simulink library "taXlibrary"  (Simulink 8.6)
settings: Solver=ode45  StartTime=0.0  StopTime=10.0  RelTol=1e-3
undefined symbols (not defined in the file): data, model, observer, scatteringDummy, sys, triJunction_12
settings Model: Creator=mur  LastModifiedBy=jaensch

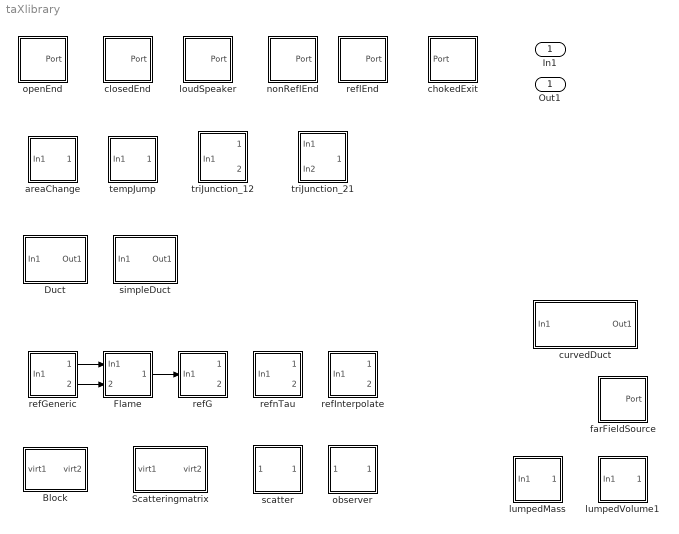
== system taXlibrary ==
  In1 : Inport
  Block : Subsystem  mask{element=Element, nIn=1, nOut=1, filename=/home/thomas/tools/taX/Projects/Orifice_Carlo/L0D_Element.mat, modelname=sys}
      mask prompts: nIn "Number of input ports"; nOut "Number of output ports"
      mask init:
      | % Set identifier
      | set_param(gcb,'element',char('Element'));
      | 
      | adaptIO(gcb);
      mask Display:
      | text(.3, .3, 'S21', 'HorizontalAlignment', 'center')
      | text(.3, .7, 'S11', 'HorizontalAlignment', 'center')
      | text(.7, .3, 'S22', 'HorizontalAlignment', 'center')
      | text(.7, .7, 'S12', 'HorizontalAlignment', 'center')
      | plot([.2 .1 .1 .2], [.9 .9 .1 .1])
      | plot([.8 .9 .9 .8], [.9 .9 .1 .1])
      | %plot([1 1 0 0 1],[1 0 0 1 1])
  Duct : Subsystem  mask{element=Duct, order=3, minres=40, l=0.5, sensorPositions=[]}
      mask prompts: order "Order of upwind scheme"; minres "Resolution of shortest wave"; l "Length [m]"; sensorPositions "Sensor Positions [m]"
      mask init:
      | % Set identifier
      | set_param(gcb,'element',char('Duct'));
      settings: AttributesFormatString=%<l> m
      mask TypeOptions order: 1 | 2 | 3 | inf
      mask Display:
      | patch([0 1 1 0],[.2 .2 .8 .8],[.7 1 1])
      | plot([0 1],[.2 .2])
      | plot([0 1],[.8 .8])
      | 
      | plot([1 1 0 0 1],[1 0 0 1 1])
  Flame : Subsystem  mask{element=rankineHugoniot, nRef=1, Mach=0.001056*101325/(287.04*293)*11.3/(101325/(287.04*1930)*0.0081*sqrt(1.4*287.04*1930)), rho=101325/(287.04*1930), c=sqrt(1.4*287.04*1930)}
      mask prompts: nRef "Number of heat release fluctuation references"; Mach "Mach number [-]"; rho "Density [Kg/m³]"; c "Speed of sound [m/s]"
      mask init:
      | set_param(gcb,'element',char('rankineHugoniot'));
      | 
      | switchNRef(gcb,nRef);
      mask Display:
      | plot([-.1 1.1], [.5 .5])
      | %patch([-.1 1.1 1.1 -.1],[-.1 -.1 1.1 1.1],[.7 1 1])
      | patch([.3 .4 .3 .4 .3 .4 .3 .4 .3 .4 .3 ...
      |        .5 .8 .5 .8 .5 .8 .5 .8 .5 .8 .5],...
      |       [ 1 .9 .8 .7 .6 .5 .4 .3 .2 .1 0 ...
      |         0 .1 .2 .3 .4 .5 .6 .7 .8 .9 1 ],[1 .75 0])
      | 
      | color('red')
      | plot([.3 .4 .3 .4 .3 .4 .3 .4 .3 .4 .3],...
      |      [ 0 .1 .2 .3 .4 .5 .6 .7 .8 .9  1])
      | plot([.4 .6 .4 .6 .4 .6 .4 .6 .4 .6 .4],...
      |      [ 0 .1 .2 .3 .4 .5 .6 .7 .8 .9  1])
      | plot([.3 .5 .8 .5 .8 .5 .8 .5 .8 .5 .8 .5 .3],...
      |      [ 0  0 .1 .2 .3 .4 .5 .6 .7 .8 .9  1  1])
  Scatteringmatrix : Subsystem  mask{element=ScatteringMatrix, filename=/home/thomas/Data/MeindlComsol/Duct/ducttest.mat, modelname=sys, l=1, A=[1], Mach=[2.2204e-18], rho=[1.3], c=[100]}
      mask prompts: l "Length [m]"; A "Area [m²]"; Mach "Mach number [-]"; rho "Density [Kg/m³]"; c "Speed of sound [m/s]"
      mask init:
      | % Set identifier
      | set_param(gcb,'element',char('ScatteringMatrix'));
      | 
      | adaptScatterIO(gcb);
      settings: AttributesFormatString=%<modelname>
      mask Display:
      | text(.3, .3, 'S21', 'HorizontalAlignment', 'center')
      | text(.3, .7, 'S11', 'HorizontalAlignment', 'center')
      | text(.7, .3, 'S22', 'HorizontalAlignment', 'center')
      | text(.7, .7, 'S12', 'HorizontalAlignment', 'center')
      | plot([.2 .1 .1 .2], [.9 .9 .1 .1])
      | plot([.8 .9 .9 .8], [.9 .9 .1 .1])
      | %plot([1 1 0 0 1],[1 0 0 1 1])
  areaChange : Subsystem  mask{element=lZeta, zeta=0, lred=0, leff=0, l=1, A=4}
      mask prompts: zeta "Pressure loss Coefficient zeta"; lred "Reduced Length l_red"; leff "Effective Length l_eff"; l "Length [m]"; A "Area [m²]"
      mask init:
      | % Set identifier
      | set_param(gcb,'element',char('lZeta'));
      settings: AttributesFormatString=%<A> m²
      mask Display:
      | patch([0 0 .6 .6  1  1 .6 .6 0], ...
      |       [.1 .9  .9 .7 .7 .3 .3  0.1 0.1], ...
      |       [.7 1 1])
      | 
      | % plot([0   0    .1 .2  .3 .4  .5 .6 .6 1   1   .6 .6  .5 .4 .3 .2  .1 0  ], ...
      | %      [ .1  .9 1   .9 1   .9 1   .9 .7  .7  .3 .3 .1 0   .1 0 .1 0    .1])
      | 
      | plot([0 .6 .6 1 1 .6 .6 0], ...
      |      [.9 .9 .7 .7 .3 .3 .1 .1])
      | 
      | plot([0 1 1 0 0], ...
      |      [1 1 0 0 1])
      | 
      | text(.3,.5,'L','HorizontalAlignment','center')
      | text(.6,.5,'zt','HorizontalAlignment','center')
  chokedExit : Subsystem  mask{element=chokedExit, loc=Downstream, Gamma=1.4, A=1, Mach=0.1, rho=1, c=100}
      mask prompts: loc "Location"; Gamma "Gamma [-]"; A "Area [m²]"; Mach "Mach number"; rho "Density [kg/m³]"; c "Speed of sound [m/s]"
      mask init:
      | % Set identifier
      | set_param(gcb,'element',char('chokedExit'));
      | 
      | switchBCUpDownStream(gcb,loc);
      mask TypeOptions loc: Downstream | Upstream
      mask Display:
      | patch([0 .5 .5 0],[.2 .2 .8 .8],[.7 1 1])
      | patch([.5 .6 .6 .5],[.2 .2 .8 .8],[.8 1 1])
      | patch([.6 .7 .7 .6],[.2 .2 .8 .8],[.9 1 1])
      | plot([0 .6 .6],[.2 .2 .35])
      | plot([0 .6 .6],[.8 .8 .65])
      | % port_label('Port',1,'M>1')
      | plot([.7 .9],[.4 .3])
      | plot([.7 .9],[.5 .5])
      | plot([.7 .9],[.6 .7])
      | plot([1 1 0 0 1],[1 0 0 1 1])
  closedEnd : Subsystem  mask{element=closedEnd, loc=Upstream, A=1, Mach=0.1, rho=1.2, c=100}
      mask prompts: loc "Location"; A "Area [m²]"; Mach "Mach number (dimensionless)"; rho "Density (Kg/m³)"; c "Speed of sound (m/s)"
      mask init:
      | if Mach<0
      |    errordlg('Mach number cannot be negative','invalid Mach number');
      | end
      | 
      | 
      | if c<=0
      |     errordlg('speed of sound must be positive','invalid speed of sound');
      | end
      | 
      | if rho<=0
      |      errordlg('density must be positive','invalid density');
      | end
      | 
      | % Set identifier
      | set_param(gcb,'element',char('closedEnd'));
      | 
      | switchBCUpDownStream(gcb,loc);
      mask TypeOptions loc: Downstream | Upstream
      mask Display:
      | plot([1 1 0 0 1],[1 0 0 1 1])
      | plot([0. .2],[.8 1.])
      | plot([0. .4],[.6 1.])
      | plot([0. .6],[.4 1.])
      | plot([0. .8],[.2 1.])
      | plot([0. 1.],[.0 1.])
      | plot([.2 1.],[.0 .8])
      | plot([.4 1.],[.0 .6])
      | plot([.6 1.],[.0 .4])
      | plot([.8 1.],[.0 .2])
  curvedDuct : Subsystem  mask{element=curvedDuct, surface_poly=exp(2.*x), d_Auto=on, d_polyin='1', n=25, l=1, A=5.184705528587072e+21}
      mask prompts: surface_poly "Area function A(x) (m²)"; d_Auto "Diameter Automatic"; d_polyin "Diameter function D(x) (m)"; n "Number of "discretization" elements"; l "Length (m)"; A "Area out (m^2)"
      mask init:
      | % Set identifier
      | set_param(gcb,'element',char('curvedDuct'));
      | 
      |    
      |    switch d_Auto
      |        case 1
      |            d_poly='-1';
      |        case 0 
      |            d_poly=d_polyin;   
      |    end
      |     
      |    tk=0;
      |    
      |   
      |    for kk = -0.5:1:n+1      
      |        tk=tk+1;
      |        xx=kk*l/n ;
      |        x=max(xx,0) ;
      |        x=min(x,l) ; 
      |        Di = double(eval(d_poly)); 
      |        switch d_Auto
      |            case 0
      |             if Di<0
      |                errordlg('diameter must be bigger than or equal to zero','invalid diameter');
      |             end
      |        end
      | 
      |        ai = double(eval(surface_poly));
      |        if ai<=0
      |            errordlg('areas must be positive','invalid areas');
      |        end
      |        d_matrix(tk,1)=Di;
      |        a_matrix(tk,1)=ai;
      |    end
      | 
      |    x = l;
      |    aj = double(eval(surface_poly));
      mask Display:
      | patch([0  .2 .3 .7 .8 1  1  .8 .7 .3 .2  0],...
      |       [.2 .1 .1 .3 .3 .2 .8 .7 .7 .9 .9 .8],[.7 1 1])
      | plot([0 .2 .3 .7 .8 1],[.2 .1 .1 .3 .3 .2])
      | plot([0 .2 .3 .7 .8 1],[.8 .9 .9 .7 .7 .8])
      | text(.4,.5,'A(x)','HorizontalAlignment','center')
      | plot([1 1 0 0 1],[1 0 0 1 1])
  farFieldSource : Subsystem  mask{element=farFieldSource, loc=Upstream, Amp=100, A=1, Mach=0.1, rho=1.2, c=100}
      mask prompts: loc "Location"; Amp "Forcing Amplitude [Pa]"; A "Area [m²]"; Mach "Mach number [-]"; rho "Density [Kg/m³]"; c "Speed of sound [m/s]"
      mask init:
      | if Mach<0
      |    errordlg('Mach number cannot be negative','invalid Mach number');
      | end
      | 
      | 
      | if c<=0
      |     errordlg('Speed of sound must be positive','invalid speed of sound');
      | end
      | 
      | if rho<=0
      |      errordlg('Density must be positive','invalid density');
      | end
      | 
      | % Set identifier
      | set_param(gcb,'element',char('farFieldSource'));
      | 
      | switchBCUpDownStream(gcb,loc);
      settings: AttributesFormatString=%<Amp> Pa
      mask TypeOptions loc: Downstream | Upstream
      mask Display:
      | patch([.55 .6  .6  .55 .45 .4  .4  .45 .55], ...
      |       [.4  .45 .55 .6  .6  .55 .45 .4  .4 ],[1 .8 .3])
      | plot([.55 .6  .6  .55 .45 .4  .4  .45 .55], ...
      |      [.4  .45 .55 .6  .6  .55 .45 .4  .4 ])
      | 
      | plot([.4  .5  .6 ],     [.65   .7  .65])
      | plot([.35 .45 .55 .65], [.75 .8 .8 .75])
      | plot([.3  .4  .6  .7 ], [.85 .9 .9 .85])
      | 
      | plot([.4  .5  .6 ],     [.35 .3 .35])
      | plot([.35 .45 .55 .65], [.25 .2 .2 .25])
      | plot([.3  .4  .6  .7 ], [.15 .1 .1 .15])
      | 
      | plot([.65 .7 .65],    [.4     .5   .6 ])
      | plot([.75 .8 .8 .75], [.35 .45 .55 .65])
      | plot([.85 .9 .9 .85], [.3  .4  .6  .7 ])
      | 
      | plot([.35 .3 .35],    [.4     .5   .6 ])
      | plot([.25 .2 .2 .25], [.35 .45 .55 .65])
      | plot([.15 .1 .1 .15], [.3  .4  .6  .7 ])
  loudSpeaker : Subsystem  mask{element=loudSpeaker, loc=Upstream, Amp=1, A=1, Mach=0.1, rho=1.2, c=100}
      mask prompts: loc "Location"; Amp "Forcing Amplitude [m/s]"; A "Area [m²]"; Mach "Mach number [-]"; rho "Density [Kg/m³]"; c "Speed of sound [m/s]"
      mask init:
      | if Mach<0
      |    errordlg('Mach number cannot be negative','invalid Mach Number');
      | end
      | 
      | 
      | if c<=0
      |     errordlg('speed of sound must be positive','invalid speed of sound');
      | end
      | 
      | if rho<=0
      |      errordlg('density must be positive','invalid density');
      | end
      | 
      | % Set identifier
      | set_param(gcb,'element',char('loudSpeaker'));
      | 
      | switchBCUpDownStream(gcb,loc);
      settings: AttributesFormatString=%<Amp> m/s
      mask TypeOptions loc: Downstream | Upstream
      mask Display:
      | switch loc
      |     case 'Upstream'
      |         patch([.2 .4 .4 .7 .7 .4 .4 .2],[.6 .6 .7 .9 .1 .3 .4 .4],[1 .8 .3])
      |         plot([.2 .2 .4 .4 .2],[.6 .4 .4 .6 .6])
      |         plot([.7 .7 .4 .4 .7],[.9 .1 .3 .7 .9])
      |     case 'Downstream'
      |         patch([.8 .6 .6 .3 .3 .6 .6 .8],[.6 .6 .7 .9 .1 .3 .4 .4],[1 .8 .3])
      |         plot([.8 .8 .6 .6 .8],[.6 .4 .4 .6 .6])
      |         plot([.3 .3 .6 .6 .3],[.9 .1 .3 .7 .9])
      | end
  lumpedMass : Subsystem  mask{element=lumpedMass, Flag=Equivalent length, Leq=1e-2, Veq=1, meq=1e-3}
      mask prompts: Flag "Form of input"; Leq "Equivalent length"; Veq "Volume"; meq "Mass"
      mask init:
      | % Set identifier
      | set_param(gcb,'element',char('lumpedMass'));
      settings: AttributesFormatString=%<Leq> m
      mask TypeOptions Flag: Equivalent length | Volume | Mass | Unflanged correction | Flanged correction
      mask Callback Flag:
      | % Get the mask parameter values. This is a cell
      | %   array of strings.
      | maskStr = get_param(gcb,'MaskValues');
      | 
      | % The pop-up menu is the first mask parameter.
      | %   Check pop-up choice by comparing first letter, i.e. E or V
      | if strcmp(maskStr{2}(1),'E'),
      |     % Turn off the visibility of V and M
      |     set_param(gcb,'MaskVisibilities',{'off';'on';'on';'off';'off'}),
      |     set_param(gcb,'MaskValues',maskStr);
      |     set_param(gcb,'AttributesFormatString',['%<Leq> m'])
      | elseif strcmp(maskStr{2}(1),'V'),
      |     % Turn off the visibility of parameters related L and M
      |     set_param(gcb,'MaskVisibilities',{'off';'on';'off';'on';'off'}),
      |     set_param(gcb,'MaskValues',maskStr);
      |     set_param(gcb,'AttributesFormatString',['%<Veq> m^3'])
      | elseif strcmp(maskStr{2}(1),'M'),
      |     % Turn off the visibility of parameters related L and V
      |     set_param(gcb,'MaskVisibilities',{'off';'on';'off';'off';'on'}),
      |     set_param(gcb,'MaskValues',maskStr);
      |     set_param(gcb,'AttributesFormatString',['%<meq> kg'])
      | else
      |     set_param(gcb,'MaskVisibilities',{'off';'on';'off';'off';'off'}),
      |     set_param(gcb,'MaskValues',maskStr);
      |     set_param(gcb,'AttributesFormatString',[maskStr{2}])
      | end
      mask Display:
      | plot([-.1 1.1],      [.5 .5])
      | 
      | patch([.3 .2 .8 .7 .3],       [.7 .2 .2 .7 .7], [.75 .75 .75])
      | plot([.3 .2 .8 .7 .5 .6 .5 .4 .5 .3],      [.7 .2 .2 .7 .7 .8 .9 .8 .7 .7])
      | text(.5,.5,'m',...
      |     'HorizontalAlignment','center')
  lumpedVolume1 : Subsystem  mask{element=lumpedVolume, Flag=Volume, Leq=1, Veq=1}
      mask prompts: Flag "Form of input"; Leq "Length"; Veq "Volume"
      mask init:
      | % Set identifier
      | set_param(gcb,'element',char('lumpedVolume'));
      settings: AttributesFormatString=%<Veq> m^3
      mask TypeOptions Flag: Equivalent length | Volume
      mask Callback Flag:
      | % Get the mask parameter values. This is a cell
      | %   array of strings.
      | maskStr = get_param(gcb,'MaskValues');
      | 
      | % The pop-up menu is the second mask parameter.
      | % Check pop-up choice by comparing first letter, i.e. E or V
      | if strcmp(maskStr{2}(1),'E'),
      |     % Turn off the visibility of V
      |     set_param(gcb,'MaskVisibilities',{'off';'on';'on';'off'});
      |     set_param(gcb,'MaskValues',maskStr);
      |     set_param(gcb,'AttributesFormatString',['%<Leq> m']);
      | else
      |     % Turn off the visibility of parameters related L
      |     set_param(gcb,'MaskVisibilities',{'off';'on';'off';'on'});
      |     set_param(gcb,'MaskValues',maskStr);
      |     set_param(gcb,'AttributesFormatString',['%<Veq> m^3']);
      | end
      mask Display:
      | patch([0 0 .1 .3 .5 .7 .9 1 ...
      |       1 .9 .7 .5 .3 .1 0], ...
      |      [.1 .9 1 .8 1 .8 1 .9 ...
      |      .1 0 .2 0 .2 0 .1],[.7 1 1])
      | 
      | plot([0 0 .1 .3 .5 .7 .9 1 ...
      |       1 .9 .7 .5 .3 .1 0], ...
      |      [.1 .9 1 .8 1 .8 1 .9 ...
      |      .1 0 .2 0 .2 0 .1])
      | 
      | disp('V')
  nonReflEnd : Subsystem  mask{element=reflEnd, loc=Upstream, r=0, A=1, Mach=0.1, rho=1.2, c=100}
      mask prompts: loc "Location"; A "Area [m²]"; Mach "Mach number (dimensionless)"; rho "Density (Kg/m³)"; c "Speed of sound (m/s)"
      mask init:
      | % Set identifier
      | set_param(gcb,'element',char('reflEnd'));
      | 
      | switchBCUpDownStream(gcb,loc);
      mask TypeOptions loc: Downstream | Upstream
      mask Display:
      | patch([0 1 1 0],[.2 .2 .8 .8],[.7 1 1])
      | 
      | %plot([0. .2],[.8 1.])
      | %plot([0. .4],[.6 1.])
      | %plot([0. .6],[.4 1.])
      | %plot([0. .8],[.2 1.])
      | %plot([0. 1.],[.0 1.])
      | %plot([.2 1.],[.0 .8])
      | %plot([.4 1.],[.0 .6])
      | %plot([.6 1.],[.0 .4])
      | %plot([.8 1.],[.0 .2])
      | 
      | plot([0.0 .05],[.2 .2])
      | plot([.15 .25],[.2 .2])
      | plot([.35 .45],[.2 .2])
      | plot([.55 .65],[.2 .2])
      | plot([.75 .85],[.2 .2])
      | plot([.95 1.0],[.2 .2])
      | 
      | plot([0.0 .05],[.8 .8])
      | plot([.15 .25],[.8 .8])
      | plot([.35 .45],[.8 .8])
      | plot([.55 .65],[.8 .8])
      | plot([.75 .85],[.8 .8])
      | plot([.95 1.0],[.8 .8])
      | 
      | plot([.2 .15 .2 .3 .4 .6 .7 .8 .85 .8 .7 .6 .4 .3 .2], ...
      |     [.4 .5 .6 .65 .6 .4 .35 .4 .5 .6 .65 .6 .4 .35 .4])
      | 
      | plot([1 1 0 0 1],[1 0 0 1 1])
  observer : Subsystem  mask{element=observer, property=p_u}
      mask prompts: property "Observed Quantity"
      mask init:
      | % Set identifier
      | set_param(gcb,'element',char('observer'));
      mask TypeOptions property: p_u | f_g
      mask Display:
      | color('red')
      | plot([0 0 1 1 0],[1 0 0 1 1])
      | 
      | plot([.5 .4 .3 .3 .4 .6 .7 .7 .4 .3 .3],[.6 .6 .7 .8 .9 .9 .7 .5 .1 .1 .2])
      | plot([.5 .4 .4 .5 .6 .65],[.6 .7 .8 .85 .8 .6])
      | plot([.4 .5 .6 .6 .5 .45 .4 .4 .45 .45 .4 .4],[.7 .7 .6 .5 .4 .3 .3 .35 .4 .45 .5 .55])
      | 
      | %plot([.9 .85 .9],    [.4     .5   .6 ])
      | %plot([.8 .75 .75 .8], [.35 .45 .55 .65])
      | 
      | %plot([.1 .15 .1],    [.4     .5   .6 ])
      | %plot([.2 .25 .25 .2], [.35 .45 .55 .65])
  openEnd : Subsystem  mask{element=openEnd, loc=Upstream, A=1, Mach=0.1, rho=1.2, c=100}
      mask prompts: loc "Location"; A "Area (m^2)"; Mach "Mach number (dimensionless)"; rho "Density (Kg/m³)"; c "Speed of sound (m/s)"
      mask init:
      | if Mach<0
      |    errordlg('Mach number cannot be negative','invalid Mach Number');
      | end
      | 
      | 
      | if c<=0
      |     errordlg('Speed of sound must be positive','invalid speed of sound');
      | end
      | 
      | if rho<=0
      |      errordlg('Density must be positive','invalid density');
      | end
      | 
      | % Set identifier
      | set_param(gcb,'element',char('openEnd'));
      | 
      | switchBCUpDownStream(gcb,loc);
      mask TypeOptions loc: Downstream | Upstream
      mask Display:
      | %patch([.2  1  1 .2],[.2 .2 .8 .8],[.7 1 1])
      | %patch([.2 .3 .3 .2],[.2 .2 .8 .8],[.9 1 1])
      | %patch([.3 .4 .4 .3],[.2 .2 .8 .8],[.8 1 1])
      | %plot([.3 1],[.2 .2])
      | %plot([.3 1],[.8 .8])
      | %plot([1 1 0 0 1],[1 0 0 1 1])
      | 
      | %patch([.2 .2 .3 .5 .6 .6 .5 .3],...
      | %      [.45 .65 .75 .75 .65 .45 .35 .35],[1 1 0])
      | color('red')
      | plot([.25 .2  .2  .3  .5  .6  .6],...
      |      [.4  .45 .65 .75 .75 .65 .5])
      | plot([.4 .4],[.85 1.0])
      | plot([-.05 .1],[.55 .55])
      | plot([.7 .85],[.55 .55])
      | plot([.2 .1],[.75 .85])
      | plot([.6 .7],[.75 .85])
      | %patch([.1 .1 .2 .4 .45 .6 .75 .9  .9 1. 1. .9 .2],...
      | %      [.1 .3 .4 .4 .35 .5  .5 .35 .3 .2 .1 .0 .0],[.7 1 1])
      | color('blue')
      | plot([ .45 .6 .75 .9  .9 1. 1. .9 .2 .1 .1 .2 .4 .6 .7],...
      |      [ .35 .5  .5 .35 .3 .2 .1 .0 .0 .1 .3 .4 .4 .2 .2])
  refG : Subsystem  mask{element=reference, filename=FTF_GFlame_Steinbacher.m, Flammentyp=V-Flame, VModell=convective, R=0.1, H=0.15, gamma=0, L1=0, L2=0, SchemeSpace=upwind, nY=50, active=on, modelname=0}
      mask prompts: Flammentyp "Flame Type"; VModell "Velocity Model"; R "Radius [m]"; H "Heigth [m]"; gamma "MFlame Gamma [m]"; L1 "MFlame L1 [m]"; L2 "MFlame L2 [m]"; SchemeSpace "Integration Scheme"; nY "Number of Discretization Points"
      mask init:
      | set_param(gcb,'element',char('reference'));
      | set_param(gcb,'filename',char('FTF_GFlame_Steinbacher.m'));
      mask TypeOptions Flammentyp: V-Flame | Conical Flame | M-Flame
      mask Callback Flammentyp:
      | % If Mflame is not selected, do not show parameters of MFlame
      | maskStr = get_param(gcb,'MaskValues');
      | 
      | if strcmp(maskStr{3}(1),'M')
      |     set_param(gcb,'MaskVisibilities',{'off';'off';'on';'on';'on';'on';'on';'on';'on';'on';'on';'on';'off'})
      | else
      |     set_param(gcb,'MaskVisibilities',{'off';'off';'on';'on';'on';'on';'off';'off';'off';'on';'on';'on';'off'})
      | end
      mask TypeOptions VModell: convective | uniform
      mask TypeOptions SchemeSpace: upwind | central
      mask Display:
      | color('red')
      | plot([0 0 1 1 0],[1 0 0 1 1])
      | 
      | plot([-1, .3, .5, 2],...
      |      [.5, .5, .8,.8])
      | 
      | port_label('output', 2, 'Ref.')
  refGeneric : Subsystem  mask{element=reference, filename=/home/thomas/tools/taX/elements/model_Luis_30kW_9.5%25.mat, modelname=model, active=on}
      mask prompts: active "Active Flame"
      mask init:
      | set_param(gcb,'element',char('reference'));
      settings: AttributesFormatString=%<modelname>
      mask Display:
      | color('red')
      | plot([0 0 1 1 0],[1 0 0 1 1])
      | 
      | plot([-1, .3, .5, 2],...
      |      [.5, .5, .8,.8])
      | 
      | port_label('output', 2, 'Ref.')
  refInterpolate : Subsystem  mask{element=reference, filename=FTF_interpolate.m, modelname=0, data=data.mat, pi=0, active=on}
      mask prompts: data "Data files"; pi "parameters"; active "Active Flame"
      mask init:
      | set_param(gcb,'element',char('reference'));
      settings: AttributesFormatString=%<modelname>
      mask Display:
      | color('red')
      | plot([0 0 1 1 0],[1 0 0 1 1])
      | 
      | plot([-1, .3, .5, 2],...
      |      [.5, .5, .8,.8])
      | 
      | port_label('output', 2, 'Ref.')
  reflEnd : Subsystem  mask{element=reflEnd, loc=Upstream, r=-0.8, A=1, Mach=0.1, rho=1.2, c=100}
      mask prompts: loc "Location"; r "Reflection coefficient"; A "Area [m²]"; Mach "Mach number [-]"; rho "Density [Kg/m³]"; c "Speed of sound [m/s]"
      mask init:
      | if Mach<0
      |    errordlg('Mach number cannot be negative','invalid Mach number');
      | end
      | 
      | 
      | if c<=0
      |     errordlg('speed of sound must be positive','invalid speed of sound');
      | end
      | 
      | 
      | if rho<=0
      |      errordlg('density must be positive','invalid density');
      | end
      | 
      | % Set identifier
      | set_param(gcb,'element',char('reflEnd'));
      | 
      | switchBCUpDownStream(gcb,loc);
      settings: AttributesFormatString=%<r>
      mask TypeOptions loc: Downstream | Upstream
      mask Display:
      | %patch([.2  1  1 .2],[.2 .2 .8 .8],[.7 1 1])
      | %patch([.2 .3 .3 .2],[.2 .2 .8 .8],[.9 1 1])
      | %patch([.3 .4 .4 .3],[.2 .2 .8 .8],[.8 1 1])
      | %plot([.25 .15],[.3 .3])
      | %plot([.25 .15],[.4 .4])
      | %plot([.25 .15],[.5 .5])
      | %plot([.25 .15],[.6 .6])
      | %plot([.25 .15],[.7 .7])
      | 
      | patch([0 1 1 0],[.2 .2 .8 .8],[.7 1 1])
      | 
      | plot([0.0 .05],[.2 .2])
      | plot([.15 .25],[.2 .2])
      | plot([.35 .45],[.2 .2])
      | plot([.55 .65],[.2 .2])
      | plot([.75 .85],[.2 .2])
      | plot([.95 1.0],[.2 .2])
      | 
      | plot([0.0 .05],[.8 .8])
      | plot([.15 .25],[.8 .8])
      | plot([.35 .45],[.8 .8])
      | plot([.55 .65],[.8 .8])
      | plot([.75 .85],[.8 .8])
      | plot([.95 1.0],[.8 .8])
      | 
      | text(.5,.5,'R','HorizontalAlignment','center')
      | 
      | %plot([.45 .55],[.7 .7])
      | %plot([.45 .55],[.6 .6])
      | %plot([.45 .55],[.5 .5])
      | %plot([.45 .55],[.4 .4])
      | %plot([.45 .55],[.3 .3])
      | plot([1 1 0 0 1],[1 0 0 1 1])
  refnTau : Subsystem  mask{element=reference, n=1, tau=1, active=on, filename=FTF_ntau.m, modelname=0}
      mask prompts: n "Interaction Index n [-]"; tau "Time delay tau [s]"; active "Active Flame"
      mask init:
      | set_param(gcb,'element',char('reference'));
      | set_param(gcb,'filename',char('FTF_ntau.m'));
      mask Display:
      | color('red')
      | plot([0 0 1 1 0],[1 0 0 1 1])
      | 
      | plot([-1, .3, .5, 2],...
      |      [.5, .5, .8,.8])
      | 
      | port_label('output', 2, 'Ref.')
  scatter : Subsystem  mask{element=scatteringDummy, loc=Upstream}
      mask prompts: loc "Location"
      mask init:
      | % Set identifier
      | set_param(gcb,'element',char('scatteringDummy'));
      mask TypeOptions loc: Downstream | Upstream
      mask Display:
      | color('red')
      | plot([0 0 1 1 0],[1 0 0 1 1])
      | 
      | switch loc
      |     case 'Upstream'
      |         plot([.35 .45 .55 .55 .45 .25 .15 .15 .45 .55 .55], ...
      |             [.6 .6 .7 .8 .9 .9 .7 .5 .1 .1 .2])
      |         plot([.35 .45 .45 .35 .25 .2],[.6 .7 .8 .85 .8 .6])
      |         plot([.45 .35 .25 .25 .35 .40 .45 .45 .40 .40 .45 .45], ...
      |             [.7 .7 .6 .5 .4 .3 .3 .35 .4 .45 .5 .55])
      | 
      |         plot([.9 .85 .9],    [.4     .5   .6 ])
      |         plot([.8 .75 .75 .8], [.35 .45 .55 .65])
      |         plot([.7 .65 .65 .7], [.3  .4  .6  .7 ])
      |     case 'Downstream'
      |         plot([.65 .55 .45 .45 .55 .75 .85 .85 .55 .45 .45], ...
      |             [.6 .6 .7 .8 .9 .9 .7 .5 .1 .1 .2])
      |         plot([.65 .55 .55 .65 .75 .8],[.6 .7 .8 .85 .8 .6])
      |         plot([.55 .65 .75 .75 .65 .6 .55 .55 .6 .6 .55 .55], ...
      |             [.7 .7 .6 .5 .4 .3 .3 .35 .4 .45 .5 .55])
      | 
      |         plot([.1 .15 .1],    [.4     .5   .6 ])
      |         plot([.2 .25 .25 .2], [.35 .45 .55 .65])
      |         plot([.3 .35 .35 .3], [.3  .4  .6  .7 ])
      | end
  simpleDuct : Subsystem  mask{element=simpleDuct, l=0.25, damping_model_popup=no damping, gm=1.4, nu=1.568e-5, Pr=5, damping_model_id=1}
      mask prompts: l "Length [m]"; damping_model_popup "Damping model"; gm "Ratio of specific heats [-]"; nu "Kinematic Viscosity [m^2/s]"; Pr "Prandtl number [-]"; damping_model_id "damping"
      mask init:
      | % Set identifier
      | set_param(gcb,'element',char('simpleDuct'));
      settings: AttributesFormatString=%<l> m
      mask TypeOptions damping_model_popup: no damping | Kirchhoff (wide tubes) | Peters | Dokumanci (best but slow) | Howe (turbulent)
      mask Callback damping_model_popup:
      | % Get the mask parameter values. This is a cell
      | %   array of strings.
      | maskStr = get_param(gcb,'MaskValues');
      | 
      | % The pop-up menu is the first mask parameter.
      | %   Check pop-up choice by comparing first letter, i.e. n or K...
      | if strcmp(maskStr{3}(1),'n'),
      |     % Turn off visibility of gamma/nu/Pr
      |     set_param(gcb,'MaskVisibilities',{'off';'on';'on';'off';'off';'off';'off'}),
      | 	maskStr{7} = '1';
      |     set_param(gcb,'MaskValues',maskStr);
      | elseif strcmp(maskStr{3}(1),'K'),
      | 	% turn on visibility of gamma/nu/Pr
      |     set_param(gcb,'MaskVisibilities',{'off';'on';'on';'on';'on';'on';'off'}),
      | 	maskStr{7} = '2';
      |     set_param(gcb,'MaskValues',maskStr);
      | elseif strcmp(maskStr{3}(1),'P'),
      | 	% turn on visibility of gamma/nu/Pr
      |     set_param(gcb,'MaskVisibilities',{'off';'on';'on';'on';'on';'on';'off'}),
      | 	maskStr{7} = '3';
      |     set_param(gcb,'MaskValues',maskStr);
      | elseif strcmp(maskStr{3}(1),'D'),
      | 	% turn on visibility of gamma/nu/Pr
      |     set_param(gcb,'MaskVisibilities',{'off';'on';'on';'on';'on';'on';'off'}),
      | 	maskStr{7} = '4';
      |     set_param(gcb,'MaskValues',maskStr);
      | else
      | 	% turn on visibility of gamma/nu
      |     set_param(gcb,'MaskVisibilities',{'off';'on';'on';'on';'on';'off';'off'}),
      | 	maskStr{7} = '5';
      |     set_param(gcb,'MaskValues',maskStr);
      | end
      mask Display:
      | patch([0 1 1 0],[.2 .2 .8 .8],[.7 1 1])
      | plot([0 1],[.2 .2])
      | plot([0 1],[.8 .8])
      | 
      | plot([1 1 0 0 1],[1 0 0 1 1])
  tempJump : Subsystem  mask{element=tempJump, Mach=694.38, rho=0.29, c=287}
      mask prompts: Mach "Mach number (dimensionless)"; rho "Density (Kg/m³)"; c "Speed of sound (m/s)"
      mask init:
      | % Set identifier
      | set_param(gcb,'element',char('tempJump'));
      mask Display:
      | %patch([-.1 1.1 1.1 -.1],[-.1 -.1 1.1 1.1],[.85 1 1])
      | text(.65,.5,'T')
      | 
      | patch([.3 .3 .2 .2 .3 .4 .5 .5 .4 .4 .3],...
      |       [.6 .4 .3 .2 .1 .1 .2 .3 .4 .6 .6], [1 0 0])
      | patch([.3 .3 .4 .4 .3],...
      |       [.9 .6 .6 .9 .9], [1 1 1])
      | plot([.3 .3 .2 .2 .3 .4 .5 .5 .4 .4 .3],...
      |      [.9 .4 .3 .2 .1 .1 .2 .3 .4 .9 .9])
      | plot([.4 .5],[.5 .5])
      | plot([.4 .5],[.6 .6])
      | plot([.4 .5],[.7 .7])
  triJunction_12 : Subsystem  mask{element=triJunction_12, zeta2=0, zeta1=0, A=[0.01  0.02]}
      mask prompts: zeta2 "Loss coefficient In1_Out2 (optional)"; zeta1 "Loss coefficient In1_Out1 (optional)"; A "Area [m²] vector"
      mask init:
      | % Set identifier
      | set_param(gcb,'element',char('triJunction_12'));
      mask DialogControl Container3 Prompt: Output properties
      mask Display:
      | %plot([0. .2],[.8 1.])
      | %plot([0. .4],[.6 1.])
      | %plot([0. .6],[.4 1.])
      | %plot([0. .8],[.2 1.])
      | %plot([0. 1.],[.0 1.])
      | %plot([.2 1.],[.0 .8])
      | %plot([.4 1.],[.0 .6])
      | %plot([.6 1.],[.0 .4])
      | %plot([.8 1.],[.0 .2])
      | 
      | patch([1 .4 0 0 .4 1 1 .6 1],[1 .8 .8 .2 .2 0 .4 .5 .6],[.7 1 1])
      | plot([1 .4 0 0 .4 1],...
      |      [1 .8 .8 .2 .2 0])
      | plot([1 1 .6 1 1],[0 .4 .5 .6 1])
      | port_label('output',1,'1')
      | port_label('output',2,'2')
      | plot([1 1 0 0 1],[1 0 0 1 1])
  triJunction_21 : Subsystem  mask{element=triJunction_21, zetai=0, zetaj=0, A=1, rho=1.2, c=100}
      mask prompts: zetai "Loss coefficient In1_Out1 (optional)"; zetaj "Loss coefficient In2_Out1 (optional)"; A "Area [m²]"; rho "Density [Kg/m³]"; c "Speed of sound [m/s]"
      mask init:
      | % Set identifier
      | set_param(gcb,'element',char('triJunction_21'));
      mask Display:
      | %plot([0. .2],[.8 1.])
      | %plot([0. .4],[.6 1.])
      | %plot([0. .6],[.4 1.])
      | %plot([0. .8],[.2 1.])
      | %plot([0. 1.],[.0 1.])
      | %plot([.2 1.],[.0 .8])
      | %plot([.4 1.],[.0 .6])
      | %plot([.6 1.],[.0 .4])
      | %plot([.8 1.],[.0 .2])
      | 
      | patch([0 .6 1   1 .6 0  0 .4  0],...
      |       [1 .8 .8 .2 .2 0 .4 .5 .6],[.7 1 1])
      | plot([0 .6 1 1 .6 0],[1 .8 .8 .2 .2 0])
      | plot([0 0 .4 0 0],[0 .4 .5 .6 1])
      | port_label('input',1,'1')
      | port_label('input',2,'2')
      | plot([1 1 0 0 1],[1 0 0 1 1])
  Out1 : Outport
  wires:
  refGeneric/2(virt1) -> Flame/2(virt1)
  refGeneric/1(Out1) -> Flame/1(In1)
  Flame/1(Out1) -> refG/1(In1)

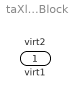
== system taXlibrary/Block ==
  virt1 : Inport
  virt2 : Outport

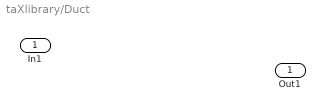
== system taXlibrary/Duct ==
  In1 : Inport
  Out1 : Outport

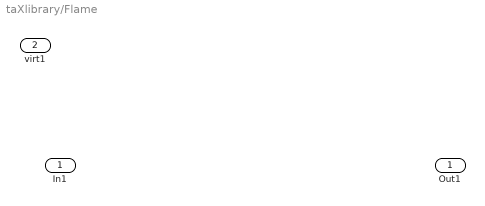
== system taXlibrary/Flame ==
  In1 : Inport
  virt1 : Inport  Port=2
  Out1 : Outport

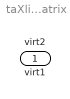
== system taXlibrary/Scatteringmatrix ==
  virt1 : Inport
  virt2 : Outport

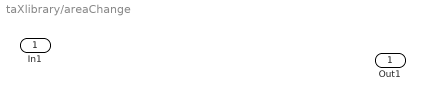
== system taXlibrary/areaChange ==
  In1 : Inport
  Out1 : Outport

== system taXlibrary/chokedExit ==
  Port : Inport

== system taXlibrary/closedEnd ==
  Port : Outport

== system taXlibrary/curvedDuct ==
  In1 : Inport
  Out1 : Outport

== system taXlibrary/farFieldSource ==
  Port : Outport

== system taXlibrary/loudSpeaker ==
  Port : Outport

== system taXlibrary/lumpedMass ==
  In1 : Inport
  Out1 : Outport

== system taXlibrary/lumpedVolume1 ==
  In1 : Inport
  Out1 : Outport

== system taXlibrary/nonReflEnd ==
  Port : Outport

== system taXlibrary/observer ==
  Port : Inport
  Port1 : Outport

== system taXlibrary/openEnd ==
  Port : Outport

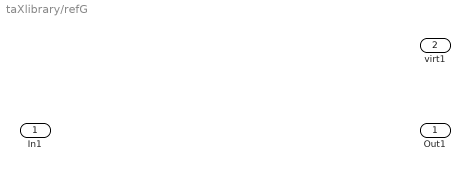
== system taXlibrary/refG ==
  In1 : Inport
  Out1 : Outport
  virt1 : Outport  Port=2

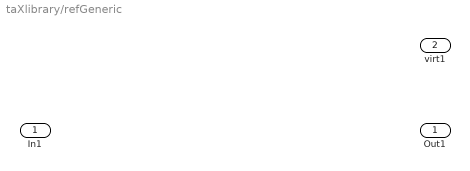
== system taXlibrary/refGeneric ==
  In1 : Inport
  Out1 : Outport
  virt1 : Outport  Port=2

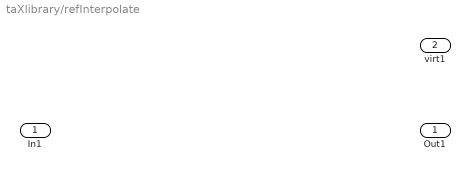
== system taXlibrary/refInterpolate ==
  In1 : Inport
  Out1 : Outport
  virt1 : Outport  Port=2

== system taXlibrary/reflEnd ==
  Port : Outport

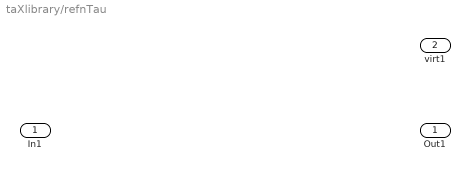
== system taXlibrary/refnTau ==
  In1 : Inport
  Out1 : Outport
  virt1 : Outport  Port=2

== system taXlibrary/scatter ==
  Port : Inport
  Port1 : Outport

== system taXlibrary/simpleDuct ==
  In1 : Inport
  Out1 : Outport

== system taXlibrary/tempJump ==
  In1 : Inport
  Out1 : Outport

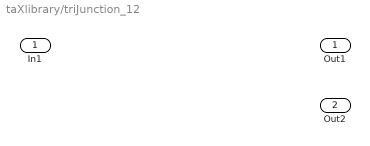
== system taXlibrary/triJunction_12 ==
  In1 : Inport
  Out1 : Outport
  Out2 : Outport  Port=2

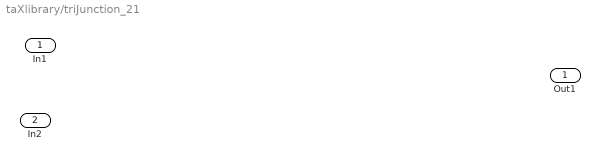
== system taXlibrary/triJunction_21 ==
  In1 : Inport
  In2 : Inport  Port=2
  Out1 : Outport
